simulink model "RefModel1"  (R2018b)
settings: Solver=VariableStepAuto  StartTime=0.0  StopTime=10.0  RelTol=1e-3
settings Model: Creator=mganesan  LastModifiedBy=mganesan

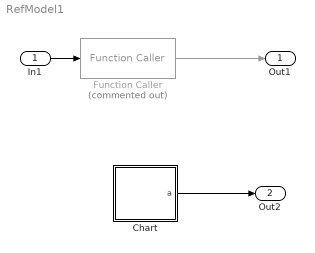
== system RefModel1 ==
  In1 : Inport
  Chart : Stateflow chart  TreatAsAtomicUnit=on
  Function Caller : FunctionCaller  Commented=on  FunctionPrototype=y = TopModel.f(u)  InputArgumentSpecifications=double(1)  OutputArgumentSpecifications=double(1)
  Out1 : Outport
  Out2 : Outport  Port=2
  wires:
  In1/1 -> Function Caller/1
  Function Caller/1 -> Out1/1
  Chart/1(a) -> Out2/1

== stateflow chart RefModel1/Chart ==
  state Init
    en:
    a=TopModel.f(1);
    a=TopModel.fnew(2);
  (default) -> Init
  data: a output double
